simulink model "Cascaded_I_PD"  (R2025a)
settings: Solver=VariableStepAuto  StartTime=0.0  StopTime=400  FixedStep=0.01  RelTol=1e-3
InitFcn:
  | parameters
values from neighbouring files (symbols this model uses):
  A = pi*(d/2)^2    (= 0.00785398163397)    [parameters.m]    (also in simulations_code.m; test.m)
  A_cross = 0.07    [parameters.m]    (also in simulations_code.m; test.m)
  C_d = 1.0    (= 1)    [parameters.m]    (also in simulations_code.m; test.m)
  d1 = 5    [parameters.m]    (also in simulation_matlab.m; simulations_code.m; test.m)
  F_pos = 2.94 + m*g    (= 32.37)    [parameters.m]    (also in sensitivity.m = 0.300 * g + m_values(i)*g; simulation_matlab.m = 2.94; simulations_code.m; test.m)
  g = 9.81    [parameters.m]    (also in simulation_matlab.m; simulations_code.m; test.m)
  k_m = 5    [parameters.m]    (also in simulation_matlab.m = 50; simulations_code.m; test.m)
  m = 3    [parameters.m]    (also in simulation_matlab.m; simulations_code.m; test.m)
  m_a = 2.5    [parameters.m]    (also in simulation_matlab.m = 0; simulations_code.m; test.m)
  p = 0.002    [parameters.m]    (also in simulation_matlab.m; simulations_code.m; test.m)
  rho = 1000    [parameters.m]    (also in simulation_matlab.m; simulations_code.m; test.m)
  V_max = 0.0005    [parameters.m]    (also in simulation_matlab.m; simulations_code.m; test.m)
  x_max = V_max / A    (= 0.0636619772368)    [parameters.m]    (also in simulations_code.m)
libraries: slpidlib x2
settings Model: Creator=hannasennero  LastModifiedBy=hannasennero
settings SolverCC: ZeroCrossAlgorithm=Adaptive
settings DebuggingCC: IgnoredZcDiagnostic=none

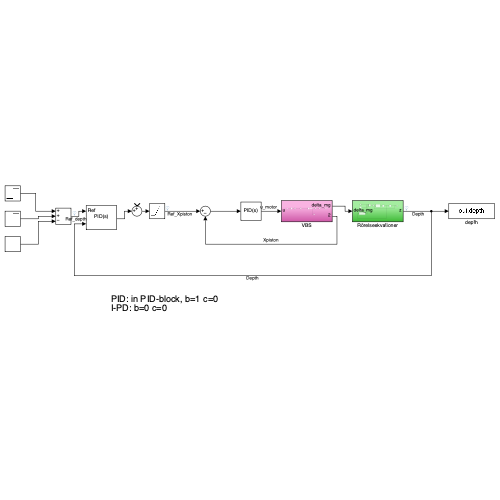
[thumbnail: Simulink's stored preview of the top-level diagram]
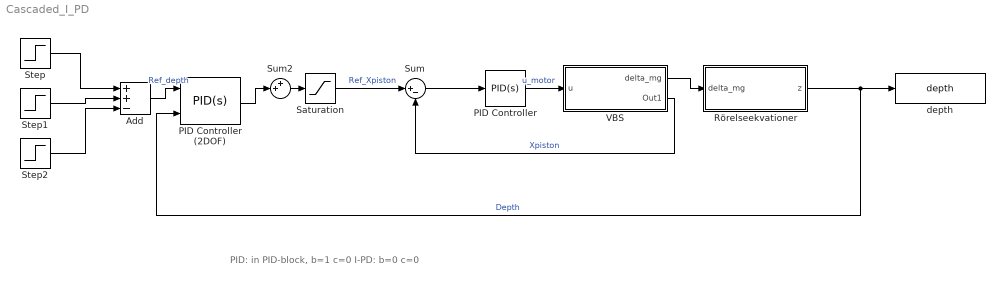
== system Cascaded_I_PD ==
  note: PID: in PID-block, b=1 c=0
      | I-PD: b=0 c=0
  Add : Sum  Inputs=++-
  PID Controller : slpidlib/PID Controller  Controller=PID  Form=Parallel  TimeDomain=Continuous-time  UseExternalTs=off  SampleTime=-1  IntegratorMethod=Forward Euler  FilterMethod=Forward Euler  ControllerParametersSource=internal  P=250  I=0  UseKiTs=off  D=0  UseExternalDerivativeSource=off  N=0  UseFilter=on  TunerSelectOption=Transfer Function Based (PID Tuner App)  InitialConditionSource=internal  InitialConditionForIntegrator=0  InitialConditionForFilter=0  DifferentiatorICPrevScaledInput=0  ExternalReset=none  TrackingMode=off  Kt=1  LimitOutput=off  SatLimitsSource=internal  UpperSaturationLimit=inf  LowerSaturationLimit=-inf  LinearizeAsGain=on  AntiWindupMode=none  Kb=1  LimitIntegrator=off  UpperIntegratorSaturationLimit=inf  LowerIntegratorSaturationLimit=-inf  POutMin=[]  POutMax=[]  IOutMin=[]  IOutMax=[]  DOutMin=[]  DOutMax=[]  NOutMin=[]  NOutMax=[]  SumOutMin=[]  SumOutMax=[]  SaturationOutMin=[]  SaturationOutMax=[]  PParamMin=[]  PParamMax=[]  IParamMin=[]  IParamMax=[]  DParamMin=[]  DParamMax=[]  NParamMin=[]  NParamMax=[]  KbParamMin=[]  KbParamMax=[]  KtParamMin=[]  KtParamMax=[]  KbOutMin=[]  KbOutMax=[]  KtOutMin=[]  KtOutMax=[]  IntegratorOutMin=[]  IntegratorOutMax=[]  FilterOutMin=[]  FilterOutMax=[]  SumI1OutMin=[]  SumI1OutMax=[]  SumI2OutMin=[]  SumI2OutMax=[]  SumI3OutMin=[]  SumI3OutMax=[]  SumI4OutMin=[]  SumI4OutMax=[]  SumDOutMin=[]  SumDOutMax=[]  DifferentiatorOutMin=[]  DifferentiatorOutMax=[]  FilterDiffOutCoefMin=[]  FilterDiffOutCoefMax=[]  ReciprocalOutMin=[]  ReciprocalOutMax=[]  SumDenOutMin=[]  SumDenOutMax=[]  SumNumOutMin=[]  SumNumOutMax=[]  DivideOutMin=[]  DivideOutMax=[]  UdiffTsProdOutMin=[]  UdiffTsProdOutMax=[]  NTsProdOutMin=[]  NTsProdOutMax=[]  UintegralTsProdOutMin=[]  UintegralTsProdOutMax=[]  UngainTsProdOutMin=[]  UngainTsProdOutMax=[]  ClampingZeroOutDataTypeStr=Inherit: Inherit via back propagation  ClampingZeroOutMin=[]  ClampingZeroOutMax=[]  FilterDenConstantOutDataTypeStr=Inherit: Inherit via back propagation  FilterDenConstantOutMin=[]  FilterDenConstantOutMax=[]  PCopyOutDataTypeStr=Inherit: Inherit via back propagation  PCopyOutMin=[]  PCopyOutMax=[]  NCopyOutDataTypeStr=Inherit: Inherit via back propagation  NCopyOutMin=[]  NCopyOutMax=[]  IntegratorContinuousStateAttributes=''  IntegratorStateMustResolveToSignalObject=off  IntegratorRTWStateStorageClass=Auto  FilterContinuousStateAttributes=''  FilterStateMustResolveToSignalObject=off  FilterRTWStateStorageClass=Auto  ParallelPVariant=InternalParameters  IdealPVariant=Disabled  IVariant=InternalParameters  DVariant=InternalParameters  IntegratorVariant=Continuous  SatVariant=Disabled  AWVariant=Passthrough  PCopyVariant=Disabled  TRVariant=Disabled  FdbkBlocksVariant=Forward  IdealPFdbkVariant=Disabled  SatFdbkVariant=Disabled  DerivativeFilterVariant=ContFilter  NVariant=InternalParameters  NCopyVariant=Disabled  FilterICVariant=InternalICsFilter  IntegratorICVariant=InternalICs  ExternalResetVariant=Disabled  TRSumVariant=Passthrough  SumFdbkVariant=Disabled  SumVariant=Sum_PID  TsampFilterVariant=InternalTs  TsampNgainVariant=Passthrough  TsampIntegralVariant=Disabled_SignalSpec  ExternalSaturationOutDataTypeStr=Inherit: Same as second input  DerivativeSourceVariant=ErrorSignal  PreIntVariant=InternalPreInt
  PID Controller (2DOF) : slpidlib/PID Controller (2DOF)  Controller=PID  Form=Parallel  TimeDomain=Continuous-time  UseExternalTs=off  SampleTime=-1  IntegratorMethod=Forward Euler  FilterMethod=Forward Euler  ControllerParametersSource=internal  P=0.008  I=0.001  UseKiTs=off  D=0.2  UseExternalDerivativeSource=off  N=0  UseFilter=on  b=0  c=0  TunerSelectOption=Transfer Function Based (PID Tuner App)  InitialConditionSource=internal  InitialConditionForIntegrator=0  InitialConditionForFilter=0  DifferentiatorICPrevScaledInput=0  ExternalReset=none  TrackingMode=off  Kt=1  LimitOutput=off  SatLimitsSource=internal  UpperSaturationLimit=inf  LowerSaturationLimit=-inf  LinearizeAsGain=on  AntiWindupMode=none  Kb=1  LimitIntegrator=off  UpperIntegratorSaturationLimit=inf  LowerIntegratorSaturationLimit=-inf  POutMin=[]  POutMax=[]  IOutMin=[]  IOutMax=[]  DOutMin=[]  DOutMax=[]  NOutMin=[]  NOutMax=[]  bOutMin=[]  bOutMax=[]  cOutMin=[]  cOutMax=[]  SumOutMin=[]  SumOutMax=[]  SaturationOutMin=[]  SaturationOutMax=[]  PParamMin=[]  PParamMax=[]  IParamMin=[]  IParamMax=[]  DParamMin=[]  DParamMax=[]  NParamMin=[]  NParamMax=[]  bParamMin=[]  bParamMax=[]  cParamMin=[]  cParamMax=[]  KbParamMin=[]  KbParamMax=[]  KtParamMin=[]  KtParamMax=[]  KbOutMin=[]  KbOutMax=[]  KtOutMin=[]  KtOutMax=[]  IntegratorOutMin=[]  IntegratorOutMax=[]  FilterOutMin=[]  FilterOutMax=[]  SumI1OutMin=[]  SumI1OutMax=[]  SumI2OutMin=[]  SumI2OutMax=[]  SumI3OutMin=[]  SumI3OutMax=[]  SumI4OutMin=[]  SumI4OutMax=[]  SumDOutMin=[]  SumDOutMax=[]  Sum1OutMin=[]  Sum1OutMax=[]  Sum2OutMin=[]  Sum2OutMax=[]  Sum3OutMin=[]  Sum3OutMax=[]  DifferentiatorOutMin=[]  DifferentiatorOutMax=[]  FilterDiffOutCoefMin=[]  FilterDiffOutCoefMax=[]  ReciprocalOutMin=[]  ReciprocalOutMax=[]  SumDenOutMin=[]  SumDenOutMax=[]  SumNumOutMin=[]  SumNumOutMax=[]  DivideOutMin=[]  DivideOutMax=[]  UdiffTsProdOutMin=[]  UdiffTsProdOutMax=[]  NTsProdOutMin=[]  NTsProdOutMax=[]  UintegralTsProdOutMin=[]  UintegralTsProdOutMax=[]  UngainTsProdOutMin=[]  UngainTsProdOutMax=[]  ClampingZeroOutDataTypeStr=Inherit: Inherit via back propagation  ClampingZeroOutMin=[]  ClampingZeroOutMax=[]  FilterDenConstantOutDataTypeStr=Inherit: Inherit via back propagation  FilterDenConstantOutMin=[]  FilterDenConstantOutMax=[]  PCopyOutDataTypeStr=Inherit: Inherit via back propagation  PCopyOutMin=[]  PCopyOutMax=[]  NCopyOutDataTypeStr=Inherit: Inherit via back propagation  NCopyOutMin=[]  NCopyOutMax=[]  IntegratorContinuousStateAttributes=''  IntegratorStateMustResolveToSignalObject=off  IntegratorRTWStateStorageClass=Auto  FilterContinuousStateAttributes=''  FilterStateMustResolveToSignalObject=off  FilterRTWStateStorageClass=Auto  ParallelPVariant=InternalParameters  IdealPVariant=Disabled  IVariant=InternalParameters  DVariant=InternalParameters  bVariant=InternalParameters  cVariant=InternalParameters  IntegratorVariant=Continuous  SatVariant=Disabled  AWVariant=Passthrough  PCopyVariant=Disabled  TRVariant=Disabled  FdbkBlocksVariant=Forward  IdealPFdbkVariant=Disabled  SatFdbkVariant=Disabled  DerivativeFilterVariant=ContFilter  NVariant=InternalParameters  NCopyVariant=Disabled  FilterICVariant=InternalICsFilter  IntegratorICVariant=InternalICs  ExternalResetVariant=Disabled  TRSumVariant=Passthrough  SumFdbkVariant=Disabled  SumVariant=Sum_PID  TsampFilterVariant=InternalTs  TsampNgainVariant=Passthrough  TsampIntegralVariant=Disabled_SignalSpec  ExternalSaturationOutDataTypeStr=Inherit: Same as second input  DerivativeSourceVariant=ErrorSignal  PreIntVariant=InternalPreInt
  Rörelseekvationer : Subsystem
  Saturation : Saturate  UpperLimit=V_max/A  LowerLimit=0
  Step : Step  After=2  SampleTime=0
  Step1 : Step  Time=100  After=5  SampleTime=0
  Step2 : Step  Time=200  After=2  SampleTime=0
  Sum : Sum  Inputs=|+-
  Sum2 : Sum  Inputs=++|
  VBS : Subsystem
  depth : ToWorkspace  VariableName=depth  SaveFormat=Timeseries  SampleTime=-1
  wires:
  Rörelseekvationer/1(z) -> PID Controller (2DOF)/2, depth/1  "Depth"
  VBS/1(delta_mg) -> Rörelseekvationer/1(delta_mg)
  PID Controller/1 -> VBS/1(u)  "u_motor"
  VBS/2(Out1) -> Sum/2  "Xpiston"
  Sum2/1 -> Saturation/1
  Saturation/1 -> Sum/1  "Ref_Xpiston"
  PID Controller (2DOF)/1 -> Sum2/2
  Sum/1 -> PID Controller/1
  Add/1 -> PID Controller (2DOF)/1  "Ref_depth"
  Step/1 -> Add/1
  Step1/1 -> Add/2
  Step2/1 -> Add/3

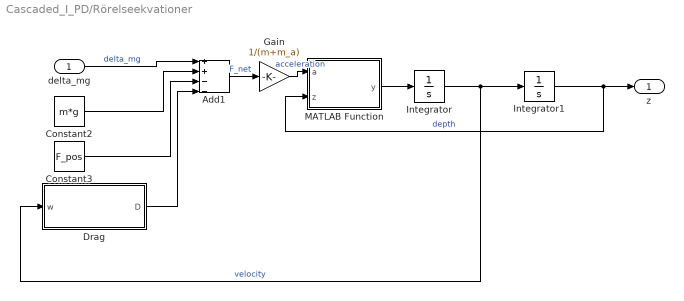
== system Cascaded_I_PD/Rörelseekvationer ==
  delta_mg : Inport
  Add1 : Sum  Inputs=++--
  Constant2 : Constant  Value=m*g
  Constant3 : Constant  Value=F_pos
  Drag : Subsystem
  Gain : Gain  Gain=1/(m+m_a)
  Integrator : Integrator  LowerSaturationLimit=0
  Integrator1 : Integrator  LimitOutput=on  LowerSaturationLimit=0
  MATLAB Function : MATLAB Function  TreatAsAtomicUnit=on
  z : Outport
  wires:
  delta_mg/1 -> Add1/1  "delta_mg"
  Constant2/1 -> Add1/2
  Constant3/1 -> Add1/3
  Drag/1(D) -> Add1/4
  Add1/1 -> Gain/1  "F_net"
  Integrator/1 -> Drag/1(w), Integrator1/1  "velocity"
  Integrator1/1 -> MATLAB Function/2(z), z/1  "depth"
  MATLAB Function/1(y) -> Integrator/1
  Gain/1 -> MATLAB Function/1(a)  "acceleration"

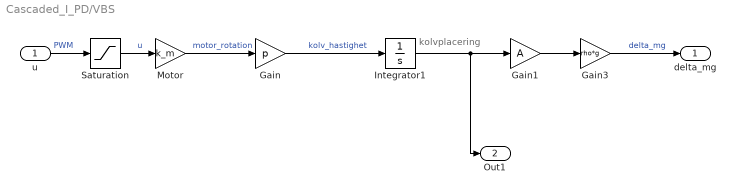
== system Cascaded_I_PD/VBS ==
  note: kolvplacering
  u : Inport
  Gain : Gain  Gain=p
  Gain1 : Gain  Gain=A
  Gain3 : Gain  Gain=rho*g
  Integrator1 : Integrator  LimitOutput=on  UpperSaturationLimit=x_max  LowerSaturationLimit=0
  Motor : Gain  Gain=k_m
  Saturation : Saturate  UpperLimit=1  LowerLimit=-1  LinearizeAsGain=off
  delta_mg : Outport
  Out1 : Outport  Port=2
  wires:
  Motor/1 -> Gain/1  "motor_rotation"
  u/1 -> Saturation/1  "PWM"
  Saturation/1 -> Motor/1  "u"
  Gain/1 -> Integrator1/1  "kolv_hastighet"
  Integrator1/1 -> Out1/1, Gain1/1
  Gain1/1 -> Gain3/1
  Gain3/1 -> delta_mg/1  "delta_mg"

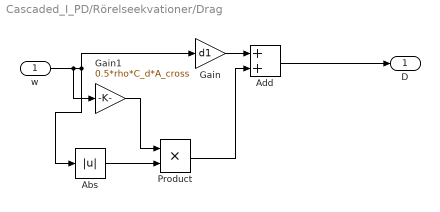
== system Cascaded_I_PD/Rörelseekvationer/Drag ==
  w : Inport
  Abs : Abs  SaturateOnIntegerOverflow=off
  Add : Sum
  Gain : Gain  Gain=d1
  Gain1 : Gain  Gain=0.5*rho*C_d*A_cross
  Product : Product
  D : Outport
  wires:
  w/1 -> Gain/1, Abs/1, Gain1/1
  Gain/1 -> Add/1
  Abs/1 -> Product/2
  Gain1/1 -> Product/1
  Product/1 -> Add/2
  Add/1 -> D/1

== matlab function Cascaded_I_PD/Rörelseekvationer/MATLAB Function ==
  data: a input; y output; z input
function y = fcn(a,z)
if a<= 0 && z <= 0
    y = 0;
else
    y = a;
end
